simulink model "generalized_energy_storage_v1"  (R2021b)
settings: Solver=VariableStepAuto  StartTime=0.0  StopTime=3600  RelTol=1e-3
InitFcn:
  | %energy storage system
  | ess.Vdc_0 = 100; %V
  | ess.Vdc_del = 50;
  | %ess.storageType = "bat"; %"sc" for supercapacitor, "bat" for battery
  | ess.storageType = "sc"; %"sc" for supercapacitor, "bat" for battery
  | 
  | ess.Ecap = 10; %total energy storage capacity, Wh
  | 
  | %determines the model parameters based on storage type, capacity, and
  | %nominal voltage
  | if ess.storageType == "bat"
  |     ess = ess_passive_bat_config(ess);
  | else %for now assume if not bat, do sc
  |     ess = ess_passive_sc_config(ess);
  | end
settings Model: Creator=jacksder  LastModifiedBy=Derek

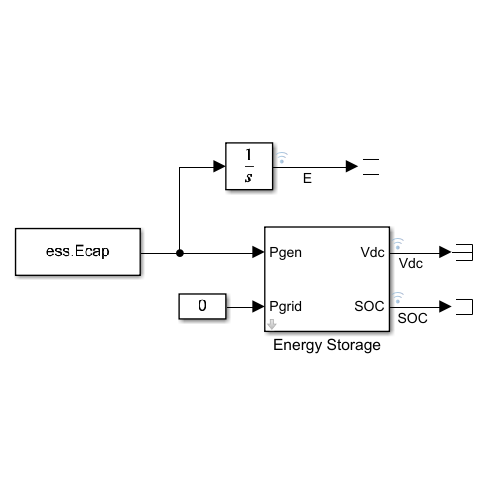
[thumbnail: Simulink's stored preview of the top-level diagram]
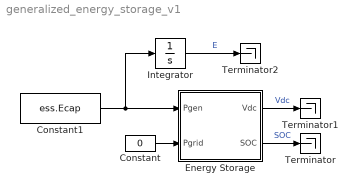
== system generalized_energy_storage_v1 ==
  Constant : Constant  Value=0
  Constant1 : Constant  Value=ess.Ecap
  Energy Storage : Subsystem  mask{SOC_0=ess.SOC_0, Csoc=ess.Csoc, SOC_LUT=ess.SOC_LUT, Voc_LUT=ess.Voc_LUT, eff=ess.eff}
      mask prompts: SOC_0 "Initial SOC"; Csoc "SOC equivalent capacitance (C):"; SOC_LUT "SOC LUT"; Voc_LUT "Voc LUT"; eff "Efficiency"
      mask DialogControl DescTextVar_copy Prompt: Uses a generalized energy storage model.
      mask DialogControl ParamGroupVar Prompt: Energy Storage Parameters
  Integrator : Integrator
  Terminator : Terminator
  Terminator1 : Terminator
  Terminator2 : Terminator
  wires:
  Constant/1 -> Energy Storage/2(Pgrid)
  Constant1/1 -> Integrator/1, Energy Storage/1(Pgen)
  Energy Storage/2(SOC) -> Terminator/1  "SOC"
  Energy Storage/1(Vdc) -> Terminator1/1  "Vdc"
  Integrator/1 -> Terminator2/1  "E"

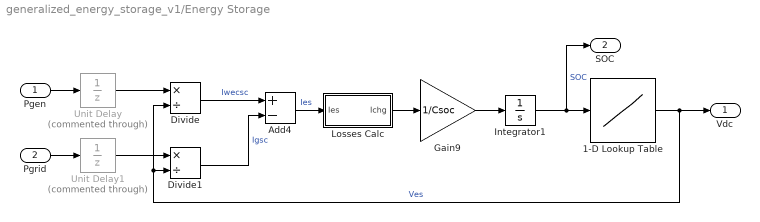
== system generalized_energy_storage_v1/Energy Storage ==
  Pgen : Inport
  Pgrid : Inport  Port=2
  1-D Lookup Table : Lookup_n-D  NumberOfTableDimensions=1  BreakpointsForDimension1=SOC_LUT  Table=Voc_LUT  InternalRulePriority=Speed  RndMeth=Simplest  InputSameDT=on
  Add4 : Sum  Inputs=+-
  Divide : Product  Inputs=*/
  Divide1 : Product  Inputs=*/
  Gain9 : Gain  Gain=1/Csoc
  Integrator1 : Integrator  InitialCondition=SOC_0
  Losses Calc : Subsystem
  Unit Delay : UnitDelay  Commented=through  SampleTime=-1  HasFrameUpgradeWarning=on
  Unit Delay1 : UnitDelay  Commented=through  SampleTime=-1  HasFrameUpgradeWarning=on
  Vdc : Outport
  SOC : Outport  Port=2
  wires:
  Unit Delay1/1 -> Divide1/1
  Unit Delay/1 -> Divide/1
  Pgrid/1 -> Unit Delay1/1
  Divide1/1 -> Add4/2  "Igsc"
  Gain9/1 -> Integrator1/1
  Divide/1 -> Add4/1  "Iwecsc"
  Pgen/1 -> Unit Delay/1
  Integrator1/1 -> SOC/1, 1-D Lookup Table/1  "SOC"
  1-D Lookup Table/1 -> Divide/2, Divide1/2, Vdc/1  "Ves"
  Add4/1 -> Losses Calc/1(Ies)  "Ies"
  Losses Calc/1(Ichg) -> Gain9/1

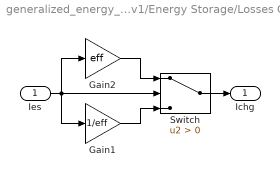
== system generalized_energy_storage_v1/Energy Storage/Losses Calc ==
  Ies : Inport
  Gain1 : Gain  Gain=1/eff
  Gain2 : Gain  Gain=eff
  Switch : Switch  Criteria=u2 > Threshold
  Ichg : Outport
  wires:
  Ies/1 -> Gain1/1, Gain2/1, Switch/2
  Switch/1 -> Ichg/1
  Gain2/1 -> Switch/1
  Gain1/1 -> Switch/3
